simulink model "LBR_MED_IK_Simul"  (R2026a)
settings: Solver=VariableStepAuto
settings Model: Creator=ivovilamowski  LastModifiedBy=ivovilamowski

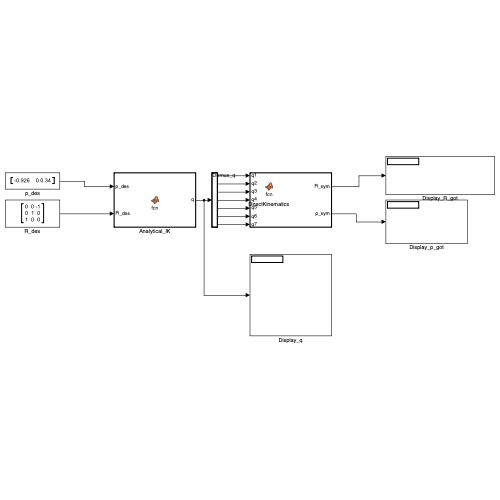
[thumbnail: Simulink's stored preview of the top-level diagram]
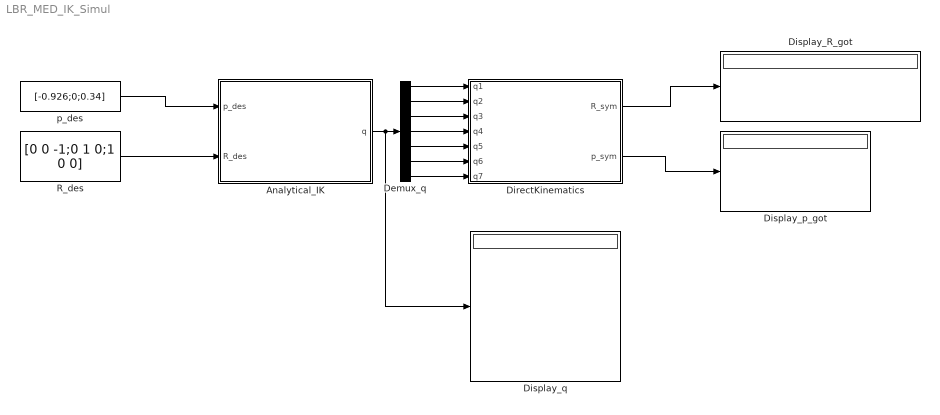
== system LBR_MED_IK_Simul ==
  Analytical_IK : MATLAB Function  TreatAsAtomicUnit=on
  Demux_q : Demux  Outputs=7
  DirectKinematics : MATLAB Function  TreatAsAtomicUnit=on
  Display_R_got : Display
  Display_p_got : Display
  Display_q : Display
  R_des : Constant  Value=[0 0 -1;0 1 0;1 0 0]
  p_des : Constant  Value=[-0.926;0;0.34]
  wires:
  p_des/1 -> Analytical_IK/1(p_des)
  R_des/1 -> Analytical_IK/2(R_des)
  Analytical_IK/1(q) -> Display_q/1, Demux_q/1
  Demux_q/1 -> DirectKinematics/1(q1)
  Demux_q/2 -> DirectKinematics/2(q2)
  Demux_q/3 -> DirectKinematics/3(q3)
  Demux_q/4 -> DirectKinematics/4(q4)
  Demux_q/5 -> DirectKinematics/5(q5)
  Demux_q/6 -> DirectKinematics/6(q6)
  Demux_q/7 -> DirectKinematics/7(q7)
  DirectKinematics/2(p_sym) -> Display_p_got/1
  DirectKinematics/1(R_sym) -> Display_R_got/1

== matlab function LBR_MED_IK_Simul/DirectKinematics ==
  data: q1 input; R_sym output; q2 input; q3 input; q4 input; q5 input; q6 input; q7 input; p_sym output
function [R_sym,p_sym] = DirectKinematics(q1,q2,q3,q4,q5,q6,q7)
%#codegen

%    This function was generated by the Symbolic Math Toolbox version 26.1.
%    12-May-2026 21:08:10

% q1 = complex(q1);  % if required to enforce complex operations
% q2 = complex(q2);  % if required to enforce complex operations
% q3 = complex(q3);  % if required to enforce complex operations
% q4 = complex(q4);  % if required to enforce complex operations
% q5 = complex(q5);  % if required to enforce complex operations
% q6 = complex(q6);  % if required to enforce complex operations
% q7 = complex(q7);  % if required to enforce complex operations
t2 = cos(q1);
t3 = cos(q2);
t4 = cos(q3);
t5 = cos(q4);
t6 = cos(q5);
t7 = cos(q6);
t8 = cos(q7);
t9 = sin(q1);
t10 = sin(q2);
t11 = sin(q3);
t12 = sin(q4);
t13 = sin(q5);
t14 = sin(q6);
t15 = sin(q7);
t16 = t2.*t4;
t17 = t3.*t5;
t18 = t2.*t11;
t19 = t4.*t9;
t20 = t3.*t12;
t21 = t9.*t11;
t22 = t9.*t10.*t12;
t23 = t10.*t11.*t13;
t27 = t2.*t5.*t10;
t28 = t4.*t5.*t10;
t30 = t2.*t10.*t12;
t31 = t5.*t9.*t10;
t32 = t4.*t10.*t12;
t33 = t6.*t10.*t11;
t24 = t3.*t16;
t25 = t3.*t18;
t26 = t3.*t19;
t29 = t3.*t21;
t35 = -t28;
t42 = t17+t32;
t34 = -t24;
t36 = -t29;
t40 = t18+t26;
t41 = t19+t25;
t45 = t20+t35;
t50 = t14.*t42;
t43 = t16+t36;
t44 = t21+t34;
t46 = t5.*t40;
t47 = t6.*t41;
t48 = t12.*t40;
t49 = t13.*t41;
t54 = t6.*t45;
t57 = t13.*t45;
t51 = t5.*t44;
t52 = t6.*t43;
t55 = t12.*t44;
t56 = t13.*t43;
t60 = t22+t46;
t62 = t23+t54;
t70 = -t14.*(t31-t48);
t63 = t27+t55;
t64 = t6.*t60;
t65 = t13.*t60;
t69 = t7.*t62;
t71 = -t6.*(t30-t51);
t68 = t14.*t63;
t73 = t56+t64;
t74 = t49+t71;
t77 = t7.*t73;
t79 = t7.*t74;
t80 = t70+t77;
t81 = t68+t79;
R_sym = reshape([-t15.*(t47+t13.*(t30-t51))-t8.*t81,t8.*t80+t15.*(t52-t65),-t15.*(t33-t57)+t8.*(t50-t69),-t8.*(t47+t13.*(t30-t51))+t15.*t81,-t15.*t80+t8.*(t52-t65),-t8.*(t33-t57)-t15.*(t50-t69),-t7.*t63+t14.*t74,-t14.*t73-t7.*(t31-t48),t7.*t42+t14.*t62],[3,3]);
if nargout > 1
    p_sym = [t27.*(-2.0./5.0)-t55.*(2.0./5.0)-t2.*t10.*(2.0./5.0)-t7.*t63.*(6.3e+1./5.0e+2)+t14.*t74.*(6.3e+1./5.0e+2);t31.*(-2.0./5.0)+t48.*(2.0./5.0)-t9.*t10.*(2.0./5.0)-t14.*t73.*(6.3e+1./5.0e+2)-t7.*(t31-t48).*(6.3e+1./5.0e+2);t3.*(2.0./5.0)+t17.*(2.0./5.0)+t32.*(2.0./5.0)+t7.*t42.*(6.3e+1./5.0e+2)+t14.*t62.*(6.3e+1./5.0e+2)+1.7e+1./5.0e+1];
end
end

== matlab function LBR_MED_IK_Simul/Analytical_IK ==
  data: p_des input; q output; R_des input
function q = ik_block(p_des, R_des)
    q = LBR_MED_IK(p_des, R_des);
end
